simulink model "Channelizer"  (R2023a)
settings: Solver=VariableStepAuto  StartTime=0.0  StopTime=inf  RelTol=1e-3
InitFcn:
  | init;
values from neighbouring files (symbols this model uses):
  ch0_en = 0    [init.m]
  ch0_qam = 0    [init.m]
  ch0_swp = 0    [init.m]
  ch10_en = 0    [init.m]
  ch10_qam = 0    [init.m]
  ch10_swp = 0    [init.m]
  ch11_en = 0    [init.m]
  ch11_qam = 0    [init.m]
  ch11_swp = 0    [init.m]
  ch12_en = 0    [init.m]
  ch12_qam = 0    [init.m]
  ch12_swp = 0    [init.m]
  ch13_en = 0    [init.m]
  ch13_qam = 0    [init.m]
  ch13_swp = 0    [init.m]
  ch14_en = 0    [init.m]
  ch14_qam = 0    [init.m]
  ch14_swp = 0    [init.m]
  ch15_en = 0    [init.m]
  ch15_qam = 0    [init.m]
  ch15_swp = 0    [init.m]
  ch1_en = 1    [init.m]
  ch1_qam = 0    [init.m]
  ch1_swp = 0    [init.m]
  ch2_en = 1    [init.m]
  ch2_qam = 0    [init.m]
  ch2_swp = 0    [init.m]
  ch3_en = 0    [init.m]
  ch3_qam = 0    [init.m]
  ch3_swp = 0    [init.m]
  ch4_en = 0    [init.m]
  ch4_qam = 0    [init.m]
  ch4_swp = 0    [init.m]
  ch5_en = 1    [init.m]
  ch5_qam = 1    [init.m]
  ch5_swp = 0    [init.m]
  ch6_en = 1    [init.m]
  ch6_qam = 1    [init.m]
  ch6_swp = 0    [init.m]
  ch7_en = 0    [init.m]
  ch7_qam = 0    [init.m]
  ch7_swp = 0    [init.m]
  ch8_en = 0    [init.m]
  ch8_qam = 0    [init.m]
  ch8_swp = 0    [init.m]
  ch9_en = 0    [init.m]
  ch9_qam = 0    [init.m]
  ch9_swp = 0    [init.m]
  ch_filt_coef = 28 * ch_filt_coef / sum(ch_filt_coef(:))    [init.m]
  N = 512    [init.m]
  spec1_ch = 1    [init.m]
  spec2_ch = 2    [init.m]
  spec3_ch = 5    [init.m]
  spec4_ch = 6    [init.m]
  swp_rate0 = 0    [init.m]
  swp_rate1 = 0    [init.m]
  swp_rate10 = 0    [init.m]
  swp_rate11 = 0    [init.m]
  swp_rate12 = 0    [init.m]
  swp_rate13 = 0    [init.m]
  swp_rate14 = 0    [init.m]
  swp_rate15 = 0    [init.m]
  swp_rate2 = 0    [init.m]
  swp_rate3 = 0    [init.m]
  swp_rate4 = 0    [init.m]
  swp_rate5 = 0    [init.m]
  swp_rate6 = 0    [init.m]
  swp_rate7 = 0    [init.m]
  swp_rate8 = 0    [init.m]
  swp_rate9 = 0    [init.m]
  Ts = 16*(7/4)/8.75e9    (= 3.2e-09)    [init.m]
undefined symbols (not defined in the file or in its folder): S, vsva2197, xcvc1902
libraries: aieBasic x56, aieUtilities x47, dspswit3 x16, dspsigops x16, hlsBasic x3, dspindex x1, vmcUtilities x1, commchan3 x1
(part 4 of 4)

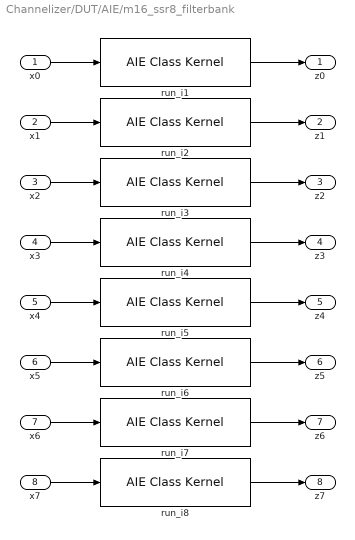
== system Channelizer/DUT/AIE/m16_ssr8_filterbank ==
  x0 : Inport
  x1 : Inport  Port=2
  x2 : Inport  Port=3
  x3 : Inport  Port=4
  x4 : Inport  Port=5
  x5 : Inport  Port=6
  x6 : Inport  Port=7
  x7 : Inport  Port=8
  run_i1 : aieBasic/AIE Class Kernel  KernelAllAttrs=|  PortNames={'sig_i'; 'sig_o'}  PortSerializedTypes={'{Q2{P{Tinput_stream{1{t{Scint16}}}}}}'; '{Q2{P{Toutput_stream{1{t{Scint16}}}}}}'}  PortWindowSizes={0.000000000000000000e+00; 0.000000000000000000e+00}  PortWindowMargins={0.000000000000000000e+00; 0.000000000000000000e+00}  PortSynchronicities={'auto', 'auto'}  PortSignalSizes={0.000000000000000000e+00; 2.048000000000000000e+03}  ClassTemplateSpecKind=implicit  ClassTemplateParamNames={'pattern'; 'NSAMP'}  ClassTemplateParamKinds={'nontype'; 'nontype'}  ClassTemplateParamTypes={'unsigned int'; 'unsigned int'}  ClassTemplateParamValues={'0', '2048'}  ClassCtorParamNames={'taps0_i'; 'taps1_i'}  ClassCtorParamSerializedTypes={'{R{C{Bi16}64}}'; '{R{C{Bi16}64}}'}  ClassCtorParamValues={'[0;2;-4;6;-13;54;-178;1985;-20;88;-287;1822;-22;100;-326;1570;2042;6;-4;2;259;-80;23;-8;569;-166;49;-9;911;-248;74;-14;-19;93;-307;1256;-14;74;-248;911;-9;49;-166;569;-8;23;-80;259;1256;-307;93;-19;1570;-326;100;-22;1822;-287;88;-20;1985;-178;54;-13]', '[6;12;-40;124;-6;28;-95;2027;-17;74;-241;1916;-22;97;-314;1706;2027;-95;28;-6;124;-40;12;6;408;-123;36;-8;737;-209;62;-12;-21;99;-322;1419;-17;85;-281;1085;-12;62;-209;737;-8;36;-123;408;1085;-281;85;-17;1419;-322;99;-21;1706;-314;97;-22;1916;-241;74;-17]'}  ClassIndex=1  ClassCtorIndex=1  ClassTabVisible=on  ClassTemplateParamsVisible=on  ClassCtorDeclVisible=on  ClassCtorParamsVisible=on  FunctionTabVisible=on  FunctionDecl=|  PortAttrs={ 'input', 'sig_i', 'input_stream_cint16 * restrict', '', '', '', ''; 'output', 'sig_o', 'output_stream_cint16 * restrict', '', '', '', '4*N' }  PortAttrsEnables={'off', 'off', 'off', 'off', 'off', 'off', 'off';'off', 'off', 'off', 'off', 'off', 'off', 'on'}  SampleTime=-1  ClassDeclTypeOptions=C[1 1]@t74@template < unsigned int pattern, unsigned int NSAMP > class polyphase_fir;  ClassDecl=template < unsigned int pattern, unsigned int NSAMP > class polyphase_fir;  ClassTemplateParams={ 'pattern', 'unsigned int', '0'; 'NSAMP', 'unsigned int', '4*N' }  ClassTemplateParamsEnables={'off', 'off', 'on';'off', 'off', 'on'}  ClassCtorDeclTypeOptions=C[1 1]@t69@polyphase_fir(int16 ( & taps0_i ) [ 64 ], int16 ( & taps1_i ) [ 64 ])  ClassCtorDecl=polyphase_fir(int16 ( & taps0_i ) [ 64 ], int16 ( & taps1_i ) [ 64 ])  ClassCtorParams={ 'taps0_i', 'int16 ( &) [ 64 ]', 'tile0_tapsA'; 'taps1_i', 'int16 ( &) [ 64 ]', 'tile0_tapsB' }  KernelHeaderFile=aie/polyphase_fir.h  KernelClassName=polyphase_fir  KernelFunction=run_i  KernelSourceFile=aie/polyphase_fir.cpp  KernelSearchPaths={}  PreProcOptions={}  blockJsonConstraints=[]
      KernelAllAttrs=|
      | s[12;12;9;9;19;14;21;23;21;23;24;21;15;17;12;24;26;26;26;27;28;9;21;23;23;23;24;25;14;19;19;29]@FunctionNameDeclFileNamePortNamesPortTypesPortSerializedTypesPortDirectionsPortWindowSizeEnablesPortWindowMarginEnablesPortBufferSizeEnablesPortBufferMarginEnablesPortSynchronicityEnablesPortSignalSizeEnablesPortBufferSizesPortBufferMarginsFunctionDeclFunctionTemplateSpecKindFunctionTemplateParamNamesFunctionTemplateParamKindsFunctionTemplateParamTypesFunctionTemplateParamValuesFunctionTemplateParamEnablesClassDeclClassTemplateSpecKindClassTemplateParamNamesClassTemplateParamKindsClassTemplateParamTypesClassTemplateParamValuesClassTemplateParamEnablesClassCtorDeclsClassCtorParamNamesClassCtorParamTypesClassCtorParamSerializedTypes[1 1]@C[32 1]@t5@run_it25@../../aie/polyphase_fir.hC[2 1]@t5@sig_it5@sig_oC[2 1]@t30@input_stream_cint16 * restrictt31@output_stream_cint16 * restrictC[2 1]@t37@{Q2{P{Tinput_stream{1{t{Scint16}}}}}}t38@{Q2{P{Toutput_stream{1{t{Scint16}}}}}}C[2 1]@t5@inputt6@outputC[2 1]@l0@l0@C[2 1]@l0@l0@C[2 1]@l0@l0@C[2 1]@l0@l0@C[2 1]@l0@l0@C[2 1]@l0@l1@C[2 1]@nnC[2 1]@nnt158@template < unsigned int pattern, unsigned int NSAMP > 
      | void polyphase_fir::
      | run_i(input_stream_cint16 * restrict sig_i, output_stream_cint16 * restrict sig_o)t4@nonee[0 1]@e[0 1]@e[0 1]@e[0 1]@e[0 1]@t74@template < unsigned int pattern, unsigned int NSAMP > class polyphase_fir;t8@implicitC[2 1]@t7@patternt5@NSAMPC[2 1]@t7@nontypet7@nontypeC[2 1]@t12@unsigned intt12@unsigned intC[2 1]@nnC[2 1]@l1@l1@C[1 1]@t69@polyphase_fir(int16 ( & taps0_i ) [ 64 ], int16 ( & taps1_i ) [ 64 ])C[1 1]@C[2 1]@t7@taps0_it7@taps1_iC[1 1]@C[2 1]@t17@int16 ( &) [ 64 ]t17@int16 ( &) [ 64 ]C[1 1]@C[2 1]@t14@{R{C{Bi16}64}}t14@{R{C{Bi16}64}}
      FunctionDecl=|
      | template < unsigned int pattern, unsigned int NSAMP > 
      | void polyphase_fir::
      | run_i(input_stream_cint16 * restrict sig_i, output_stream_cint16 * restrict sig_o)
  run_i2 : aieBasic/AIE Class Kernel  KernelAllAttrs=|  PortNames={'sig_i'; 'sig_o'}  PortSerializedTypes={'{Q2{P{Tinput_stream{1{t{Scint16}}}}}}'; '{Q2{P{Toutput_stream{1{t{Scint16}}}}}}'}  PortWindowSizes={0.000000000000000000e+00; 0.000000000000000000e+00}  PortWindowMargins={0.000000000000000000e+00; 0.000000000000000000e+00}  PortSynchronicities={'auto', 'auto'}  PortSignalSizes={0.000000000000000000e+00; 2.048000000000000000e+03}  ClassTemplateSpecKind=implicit  ClassTemplateParamNames={'pattern'; 'NSAMP'}  ClassTemplateParamKinds={'nontype'; 'nontype'}  ClassTemplateParamTypes={'unsigned int'; 'unsigned int'}  ClassTemplateParamValues={'1', '2048'}  ClassCtorParamNames={'taps0_i'; 'taps1_i'}  ClassCtorParamSerializedTypes={'{R{C{Bi16}64}}'; '{R{C{Bi16}64}}'}  ClassCtorParamValues={'[-8;23;-80;259;0;2;-4;6;-13;54;-178;1985;-20;88;-287;1822;1985;-178;54;-13;2042;6;-4;2;259;-80;23;-8;569;-166;49;-9;-22;100;-326;1570;-19;93;-307;1256;-14;74;-248;911;-9;49;-166;569;911;-248;74;-14;1256;-307;93;-19;1570;-326;100;-22;1822;-287;88;-20]', '[-8;36;-123;408;6;12;-40;124;-6;28;-95;2027;-17;74;-241;1916;1916;-241;74;-17;2027;-95;28;-6;124;-40;12;6;408;-123;36;-8;-22;97;-314;1706;-21;99;-322;1419;-17;85;-281;1085;-12;62;-209;737;737;-209;62;-12;1085;-281;85;-17;1419;-322;99;-21;1706;-314;97;-22]'}  ClassIndex=1  ClassCtorIndex=1  ClassTabVisible=on  ClassTemplateParamsVisible=on  ClassCtorDeclVisible=on  ClassCtorParamsVisible=on  FunctionTabVisible=on  FunctionDecl=|  PortAttrs={ 'input', 'sig_i', 'input_stream_cint16 * restrict', '', '', '', ''; 'output', 'sig_o', 'output_stream_cint16 * restrict', '', '', '', '4*N' }  PortAttrsEnables={'off', 'off', 'off', 'off', 'off', 'off', 'off';'off', 'off', 'off', 'off', 'off', 'off', 'on'}  SampleTime=-1  ClassDeclTypeOptions=C[1 1]@t74@template < unsigned int pattern, unsigned int NSAMP > class polyphase_fir;  ClassDecl=template < unsigned int pattern, unsigned int NSAMP > class polyphase_fir;  ClassTemplateParams={ 'pattern', 'unsigned int', '1'; 'NSAMP', 'unsigned int', '4*N' }  ClassTemplateParamsEnables={'off', 'off', 'on';'off', 'off', 'on'}  ClassCtorDeclTypeOptions=C[1 1]@t69@polyphase_fir(int16 ( & taps0_i ) [ 64 ], int16 ( & taps1_i ) [ 64 ])  ClassCtorDecl=polyphase_fir(int16 ( & taps0_i ) [ 64 ], int16 ( & taps1_i ) [ 64 ])  ClassCtorParams={ 'taps0_i', 'int16 ( &) [ 64 ]', 'tile1_tapsA'; 'taps1_i', 'int16 ( &) [ 64 ]', 'tile1_tapsB' }  KernelHeaderFile=aie/polyphase_fir.h  KernelClassName=polyphase_fir  KernelFunction=run_i  KernelSourceFile=aie/polyphase_fir.cpp  KernelSearchPaths={}  PreProcOptions={}  blockJsonConstraints=[]
      KernelAllAttrs=|
      | s[12;12;9;9;19;14;21;23;21;23;24;21;15;17;12;24;26;26;26;27;28;9;21;23;23;23;24;25;14;19;19;29]@FunctionNameDeclFileNamePortNamesPortTypesPortSerializedTypesPortDirectionsPortWindowSizeEnablesPortWindowMarginEnablesPortBufferSizeEnablesPortBufferMarginEnablesPortSynchronicityEnablesPortSignalSizeEnablesPortBufferSizesPortBufferMarginsFunctionDeclFunctionTemplateSpecKindFunctionTemplateParamNamesFunctionTemplateParamKindsFunctionTemplateParamTypesFunctionTemplateParamValuesFunctionTemplateParamEnablesClassDeclClassTemplateSpecKindClassTemplateParamNamesClassTemplateParamKindsClassTemplateParamTypesClassTemplateParamValuesClassTemplateParamEnablesClassCtorDeclsClassCtorParamNamesClassCtorParamTypesClassCtorParamSerializedTypes[1 1]@C[32 1]@t5@run_it25@../../aie/polyphase_fir.hC[2 1]@t5@sig_it5@sig_oC[2 1]@t30@input_stream_cint16 * restrictt31@output_stream_cint16 * restrictC[2 1]@t37@{Q2{P{Tinput_stream{1{t{Scint16}}}}}}t38@{Q2{P{Toutput_stream{1{t{Scint16}}}}}}C[2 1]@t5@inputt6@outputC[2 1]@l0@l0@C[2 1]@l0@l0@C[2 1]@l0@l0@C[2 1]@l0@l0@C[2 1]@l0@l0@C[2 1]@l0@l1@C[2 1]@nnC[2 1]@nnt158@template < unsigned int pattern, unsigned int NSAMP > 
      | void polyphase_fir::
      | run_i(input_stream_cint16 * restrict sig_i, output_stream_cint16 * restrict sig_o)t4@nonee[0 1]@e[0 1]@e[0 1]@e[0 1]@e[0 1]@t74@template < unsigned int pattern, unsigned int NSAMP > class polyphase_fir;t8@implicitC[2 1]@t7@patternt5@NSAMPC[2 1]@t7@nontypet7@nontypeC[2 1]@t12@unsigned intt12@unsigned intC[2 1]@nnC[2 1]@l1@l1@C[1 1]@t69@polyphase_fir(int16 ( & taps0_i ) [ 64 ], int16 ( & taps1_i ) [ 64 ])C[1 1]@C[2 1]@t7@taps0_it7@taps1_iC[1 1]@C[2 1]@t17@int16 ( &) [ 64 ]t17@int16 ( &) [ 64 ]C[1 1]@C[2 1]@t14@{R{C{Bi16}64}}t14@{R{C{Bi16}64}}
      FunctionDecl=|
      | template < unsigned int pattern, unsigned int NSAMP > 
      | void polyphase_fir::
      | run_i(input_stream_cint16 * restrict sig_i, output_stream_cint16 * restrict sig_o)
  run_i3 : aieBasic/AIE Class Kernel  KernelAllAttrs=|  PortNames={'sig_i'; 'sig_o'}  PortSerializedTypes={'{Q2{P{Tinput_stream{1{t{Scint16}}}}}}'; '{Q2{P{Toutput_stream{1{t{Scint16}}}}}}'}  PortWindowSizes={0.000000000000000000e+00; 0.000000000000000000e+00}  PortWindowMargins={0.000000000000000000e+00; 0.000000000000000000e+00}  PortSynchronicities={'auto', 'auto'}  PortSignalSizes={0.000000000000000000e+00; 2.048000000000000000e+03}  ClassTemplateSpecKind=implicit  ClassTemplateParamNames={'pattern'; 'NSAMP'}  ClassTemplateParamKinds={'nontype'; 'nontype'}  ClassTemplateParamTypes={'unsigned int'; 'unsigned int'}  ClassTemplateParamValues={'2', '2048'}  ClassCtorParamNames={'taps0_i'; 'taps1_i'}  ClassCtorParamSerializedTypes={'{R{C{Bi16}64}}'; '{R{C{Bi16}64}}'}  ClassCtorParamValues={'[-9;49;-166;569;-8;23;-80;259;0;2;-4;6;-13;54;-178;1985;1822;-287;88;-20;1985;-178;54;-13;2042;6;-4;2;259;-80;23;-8;-20;88;-287;1822;-22;100;-326;1570;-19;93;-307;1256;-14;74;-248;911;569;-166;49;-9;911;-248;74;-14;1256;-307;93;-19;1570;-326;100;-22]', '[-12;62;-209;737;-8;36;-123;408;6;12;-40;124;-6;28;-95;2027;1706;-314;97;-22;1916;-241;74;-17;2027;-95;28;-6;124;-40;12;6;-17;74;-241;1916;-22;97;-314;1706;-21;99;-322;1419;-17;85;-281;1085;408;-123;36;-8;737;-209;62;-12;1085;-281;85;-17;1419;-322;99;-21]'}  ClassIndex=1  ClassCtorIndex=1  ClassTabVisible=on  ClassTemplateParamsVisible=on  ClassCtorDeclVisible=on  ClassCtorParamsVisible=on  FunctionTabVisible=on  FunctionDecl=|  PortAttrs={ 'input', 'sig_i', 'input_stream_cint16 * restrict', '', '', '', ''; 'output', 'sig_o', 'output_stream_cint16 * restrict', '', '', '', '4*N' }  PortAttrsEnables={'off', 'off', 'off', 'off', 'off', 'off', 'off';'off', 'off', 'off', 'off', 'off', 'off', 'on'}  SampleTime=-1  ClassDeclTypeOptions=C[1 1]@t74@template < unsigned int pattern, unsigned int NSAMP > class polyphase_fir;  ClassDecl=template < unsigned int pattern, unsigned int NSAMP > class polyphase_fir;  ClassTemplateParams={ 'pattern', 'unsigned int', '2'; 'NSAMP', 'unsigned int', '4*N' }  ClassTemplateParamsEnables={'off', 'off', 'on';'off', 'off', 'on'}  ClassCtorDeclTypeOptions=C[1 1]@t69@polyphase_fir(int16 ( & taps0_i ) [ 64 ], int16 ( & taps1_i ) [ 64 ])  ClassCtorDecl=polyphase_fir(int16 ( & taps0_i ) [ 64 ], int16 ( & taps1_i ) [ 64 ])  ClassCtorParams={ 'taps0_i', 'int16 ( &) [ 64 ]', 'tile2_tapsA'; 'taps1_i', 'int16 ( &) [ 64 ]', 'tile2_tapsB' }  KernelHeaderFile=aie/polyphase_fir.h  KernelClassName=polyphase_fir  KernelFunction=run_i  KernelSourceFile=aie/polyphase_fir.cpp  KernelSearchPaths={}  PreProcOptions={}  blockJsonConstraints=[]
      KernelAllAttrs=|
      | s[12;12;9;9;19;14;21;23;21;23;24;21;15;17;12;24;26;26;26;27;28;9;21;23;23;23;24;25;14;19;19;29]@FunctionNameDeclFileNamePortNamesPortTypesPortSerializedTypesPortDirectionsPortWindowSizeEnablesPortWindowMarginEnablesPortBufferSizeEnablesPortBufferMarginEnablesPortSynchronicityEnablesPortSignalSizeEnablesPortBufferSizesPortBufferMarginsFunctionDeclFunctionTemplateSpecKindFunctionTemplateParamNamesFunctionTemplateParamKindsFunctionTemplateParamTypesFunctionTemplateParamValuesFunctionTemplateParamEnablesClassDeclClassTemplateSpecKindClassTemplateParamNamesClassTemplateParamKindsClassTemplateParamTypesClassTemplateParamValuesClassTemplateParamEnablesClassCtorDeclsClassCtorParamNamesClassCtorParamTypesClassCtorParamSerializedTypes[1 1]@C[32 1]@t5@run_it25@../../aie/polyphase_fir.hC[2 1]@t5@sig_it5@sig_oC[2 1]@t30@input_stream_cint16 * restrictt31@output_stream_cint16 * restrictC[2 1]@t37@{Q2{P{Tinput_stream{1{t{Scint16}}}}}}t38@{Q2{P{Toutput_stream{1{t{Scint16}}}}}}C[2 1]@t5@inputt6@outputC[2 1]@l0@l0@C[2 1]@l0@l0@C[2 1]@l0@l0@C[2 1]@l0@l0@C[2 1]@l0@l0@C[2 1]@l0@l1@C[2 1]@nnC[2 1]@nnt158@template < unsigned int pattern, unsigned int NSAMP > 
      | void polyphase_fir::
      | run_i(input_stream_cint16 * restrict sig_i, output_stream_cint16 * restrict sig_o)t4@nonee[0 1]@e[0 1]@e[0 1]@e[0 1]@e[0 1]@t74@template < unsigned int pattern, unsigned int NSAMP > class polyphase_fir;t8@implicitC[2 1]@t7@patternt5@NSAMPC[2 1]@t7@nontypet7@nontypeC[2 1]@t12@unsigned intt12@unsigned intC[2 1]@nnC[2 1]@l1@l1@C[1 1]@t69@polyphase_fir(int16 ( & taps0_i ) [ 64 ], int16 ( & taps1_i ) [ 64 ])C[1 1]@C[2 1]@t7@taps0_it7@taps1_iC[1 1]@C[2 1]@t17@int16 ( &) [ 64 ]t17@int16 ( &) [ 64 ]C[1 1]@C[2 1]@t14@{R{C{Bi16}64}}t14@{R{C{Bi16}64}}
      FunctionDecl=|
      | template < unsigned int pattern, unsigned int NSAMP > 
      | void polyphase_fir::
      | run_i(input_stream_cint16 * restrict sig_i, output_stream_cint16 * restrict sig_o)
  run_i4 : aieBasic/AIE Class Kernel  KernelAllAttrs=|  PortNames={'sig_i'; 'sig_o'}  PortSerializedTypes={'{Q2{P{Tinput_stream{1{t{Scint16}}}}}}'; '{Q2{P{Toutput_stream{1{t{Scint16}}}}}}'}  PortWindowSizes={0.000000000000000000e+00; 0.000000000000000000e+00}  PortWindowMargins={0.000000000000000000e+00; 0.000000000000000000e+00}  PortSynchronicities={'auto', 'auto'}  PortSignalSizes={0.000000000000000000e+00; 2.048000000000000000e+03}  ClassTemplateSpecKind=implicit  ClassTemplateParamNames={'pattern'; 'NSAMP'}  ClassTemplateParamKinds={'nontype'; 'nontype'}  ClassTemplateParamTypes={'unsigned int'; 'unsigned int'}  ClassTemplateParamValues={'3', '2048'}  ClassCtorParamNames={'taps0_i'; 'taps1_i'}  ClassCtorParamSerializedTypes={'{R{C{Bi16}64}}'; '{R{C{Bi16}64}}'}  ClassCtorParamValues={'[-14;74;-248;911;-9;49;-166;569;-8;23;-80;259;0;2;-4;6;1570;-326;100;-22;1822;-287;88;-20;1985;-178;54;-13;2042;6;-4;2;-13;54;-178;1985;-20;88;-287;1822;-22;100;-326;1570;-19;93;-307;1256;259;-80;23;-8;569;-166;49;-9;911;-248;74;-14;1256;-307;93;-19]', '[-17;85;-281;1085;-12;62;-209;737;-8;36;-123;408;6;12;-40;124;1419;-322;99;-21;1706;-314;97;-22;1916;-241;74;-17;2027;-95;28;-6;-6;28;-95;2027;-17;74;-241;1916;-22;97;-314;1706;-21;99;-322;1419;124;-40;12;6;408;-123;36;-8;737;-209;62;-12;1085;-281;85;-17]'}  ClassIndex=1  ClassCtorIndex=1  ClassTabVisible=on  ClassTemplateParamsVisible=on  ClassCtorDeclVisible=on  ClassCtorParamsVisible=on  FunctionTabVisible=on  FunctionDecl=|  PortAttrs={ 'input', 'sig_i', 'input_stream_cint16 * restrict', '', '', '', ''; 'output', 'sig_o', 'output_stream_cint16 * restrict', '', '', '', '4*N' }  PortAttrsEnables={'off', 'off', 'off', 'off', 'off', 'off', 'off';'off', 'off', 'off', 'off', 'off', 'off', 'on'}  SampleTime=-1  ClassDeclTypeOptions=C[1 1]@t74@template < unsigned int pattern, unsigned int NSAMP > class polyphase_fir;  ClassDecl=template < unsigned int pattern, unsigned int NSAMP > class polyphase_fir;  ClassTemplateParams={ 'pattern', 'unsigned int', '3'; 'NSAMP', 'unsigned int', '4*N' }  ClassTemplateParamsEnables={'off', 'off', 'on';'off', 'off', 'on'}  ClassCtorDeclTypeOptions=C[1 1]@t69@polyphase_fir(int16 ( & taps0_i ) [ 64 ], int16 ( & taps1_i ) [ 64 ])  ClassCtorDecl=polyphase_fir(int16 ( & taps0_i ) [ 64 ], int16 ( & taps1_i ) [ 64 ])  ClassCtorParams={ 'taps0_i', 'int16 ( &) [ 64 ]', 'tile3_tapsA'; 'taps1_i', 'int16 ( &) [ 64 ]', 'tile3_tapsB' }  KernelHeaderFile=aie/polyphase_fir.h  KernelClassName=polyphase_fir  KernelFunction=run_i  KernelSourceFile=aie/polyphase_fir.cpp  KernelSearchPaths={}  PreProcOptions={}  blockJsonConstraints=[]
      KernelAllAttrs=|
      | s[12;12;9;9;19;14;21;23;21;23;24;21;15;17;12;24;26;26;26;27;28;9;21;23;23;23;24;25;14;19;19;29]@FunctionNameDeclFileNamePortNamesPortTypesPortSerializedTypesPortDirectionsPortWindowSizeEnablesPortWindowMarginEnablesPortBufferSizeEnablesPortBufferMarginEnablesPortSynchronicityEnablesPortSignalSizeEnablesPortBufferSizesPortBufferMarginsFunctionDeclFunctionTemplateSpecKindFunctionTemplateParamNamesFunctionTemplateParamKindsFunctionTemplateParamTypesFunctionTemplateParamValuesFunctionTemplateParamEnablesClassDeclClassTemplateSpecKindClassTemplateParamNamesClassTemplateParamKindsClassTemplateParamTypesClassTemplateParamValuesClassTemplateParamEnablesClassCtorDeclsClassCtorParamNamesClassCtorParamTypesClassCtorParamSerializedTypes[1 1]@C[32 1]@t5@run_it25@../../aie/polyphase_fir.hC[2 1]@t5@sig_it5@sig_oC[2 1]@t30@input_stream_cint16 * restrictt31@output_stream_cint16 * restrictC[2 1]@t37@{Q2{P{Tinput_stream{1{t{Scint16}}}}}}t38@{Q2{P{Toutput_stream{1{t{Scint16}}}}}}C[2 1]@t5@inputt6@outputC[2 1]@l0@l0@C[2 1]@l0@l0@C[2 1]@l0@l0@C[2 1]@l0@l0@C[2 1]@l0@l0@C[2 1]@l0@l1@C[2 1]@nnC[2 1]@nnt158@template < unsigned int pattern, unsigned int NSAMP > 
      | void polyphase_fir::
      | run_i(input_stream_cint16 * restrict sig_i, output_stream_cint16 * restrict sig_o)t4@nonee[0 1]@e[0 1]@e[0 1]@e[0 1]@e[0 1]@t74@template < unsigned int pattern, unsigned int NSAMP > class polyphase_fir;t8@implicitC[2 1]@t7@patternt5@NSAMPC[2 1]@t7@nontypet7@nontypeC[2 1]@t12@unsigned intt12@unsigned intC[2 1]@nnC[2 1]@l1@l1@C[1 1]@t69@polyphase_fir(int16 ( & taps0_i ) [ 64 ], int16 ( & taps1_i ) [ 64 ])C[1 1]@C[2 1]@t7@taps0_it7@taps1_iC[1 1]@C[2 1]@t17@int16 ( &) [ 64 ]t17@int16 ( &) [ 64 ]C[1 1]@C[2 1]@t14@{R{C{Bi16}64}}t14@{R{C{Bi16}64}}
      FunctionDecl=|
      | template < unsigned int pattern, unsigned int NSAMP > 
      | void polyphase_fir::
      | run_i(input_stream_cint16 * restrict sig_i, output_stream_cint16 * restrict sig_o)
  run_i5 : aieBasic/AIE Class Kernel  KernelAllAttrs=|  PortNames={'sig_i'; 'sig_o'}  PortSerializedTypes={'{Q2{P{Tinput_stream{1{t{Scint16}}}}}}'; '{Q2{P{Toutput_stream{1{t{Scint16}}}}}}'}  PortWindowSizes={0.000000000000000000e+00; 0.000000000000000000e+00}  PortWindowMargins={0.000000000000000000e+00; 0.000000000000000000e+00}  PortSynchronicities={'auto', 'auto'}  PortSignalSizes={0.000000000000000000e+00; 2.048000000000000000e+03}  ClassTemplateSpecKind=implicit  ClassTemplateParamNames={'pattern'; 'NSAMP'}  ClassTemplateParamKinds={'nontype'; 'nontype'}  ClassTemplateParamTypes={'unsigned int'; 'unsigned int'}  ClassTemplateParamValues={'4', '2048'}  ClassCtorParamNames={'taps0_i'; 'taps1_i'}  ClassCtorParamSerializedTypes={'{R{C{Bi16}64}}'; '{R{C{Bi16}64}}'}  ClassCtorParamValues={'[-19;93;-307;1256;-14;74;-248;911;-9;49;-166;569;-8;23;-80;259;1256;-307;93;-19;1570;-326;100;-22;1822;-287;88;-20;1985;-178;54;-13;0;2;-4;6;-13;54;-178;1985;-20;88;-287;1822;-22;100;-326;1570;2042;6;-4;2;259;-80;23;-8;569;-166;49;-9;911;-248;74;-14]', '[-21;99;-322;1419;-17;85;-281;1085;-12;62;-209;737;-8;36;-123;408;1085;-281;85;-17;1419;-322;99;-21;1706;-314;97;-22;1916;-241;74;-17;6;12;-40;124;-6;28;-95;2027;-17;74;-241;1916;-22;97;-314;1706;2027;-95;28;-6;124;-40;12;6;408;-123;36;-8;737;-209;62;-12]'}  ClassIndex=1  ClassCtorIndex=1  ClassTabVisible=on  ClassTemplateParamsVisible=on  ClassCtorDeclVisible=on  ClassCtorParamsVisible=on  FunctionTabVisible=on  FunctionDecl=|  PortAttrs={ 'input', 'sig_i', 'input_stream_cint16 * restrict', '', '', '', ''; 'output', 'sig_o', 'output_stream_cint16 * restrict', '', '', '', '4*N' }  PortAttrsEnables={'off', 'off', 'off', 'off', 'off', 'off', 'off';'off', 'off', 'off', 'off', 'off', 'off', 'on'}  SampleTime=-1  ClassDeclTypeOptions=C[1 1]@t74@template < unsigned int pattern, unsigned int NSAMP > class polyphase_fir;  ClassDecl=template < unsigned int pattern, unsigned int NSAMP > class polyphase_fir;  ClassTemplateParams={ 'pattern', 'unsigned int', '4'; 'NSAMP', 'unsigned int', '4*N' }  ClassTemplateParamsEnables={'off', 'off', 'on';'off', 'off', 'on'}  ClassCtorDeclTypeOptions=C[1 1]@t69@polyphase_fir(int16 ( & taps0_i ) [ 64 ], int16 ( & taps1_i ) [ 64 ])  ClassCtorDecl=polyphase_fir(int16 ( & taps0_i ) [ 64 ], int16 ( & taps1_i ) [ 64 ])  ClassCtorParams={ 'taps0_i', 'int16 ( &) [ 64 ]', 'tile4_tapsA'; 'taps1_i', 'int16 ( &) [ 64 ]', 'tile4_tapsB' }  KernelHeaderFile=aie/polyphase_fir.h  KernelClassName=polyphase_fir  KernelFunction=run_i  KernelSourceFile=aie/polyphase_fir.cpp  KernelSearchPaths={}  PreProcOptions={}  blockJsonConstraints=[]
      KernelAllAttrs=|
      | s[12;12;9;9;19;14;21;23;21;23;24;21;15;17;12;24;26;26;26;27;28;9;21;23;23;23;24;25;14;19;19;29]@FunctionNameDeclFileNamePortNamesPortTypesPortSerializedTypesPortDirectionsPortWindowSizeEnablesPortWindowMarginEnablesPortBufferSizeEnablesPortBufferMarginEnablesPortSynchronicityEnablesPortSignalSizeEnablesPortBufferSizesPortBufferMarginsFunctionDeclFunctionTemplateSpecKindFunctionTemplateParamNamesFunctionTemplateParamKindsFunctionTemplateParamTypesFunctionTemplateParamValuesFunctionTemplateParamEnablesClassDeclClassTemplateSpecKindClassTemplateParamNamesClassTemplateParamKindsClassTemplateParamTypesClassTemplateParamValuesClassTemplateParamEnablesClassCtorDeclsClassCtorParamNamesClassCtorParamTypesClassCtorParamSerializedTypes[1 1]@C[32 1]@t5@run_it25@../../aie/polyphase_fir.hC[2 1]@t5@sig_it5@sig_oC[2 1]@t30@input_stream_cint16 * restrictt31@output_stream_cint16 * restrictC[2 1]@t37@{Q2{P{Tinput_stream{1{t{Scint16}}}}}}t38@{Q2{P{Toutput_stream{1{t{Scint16}}}}}}C[2 1]@t5@inputt6@outputC[2 1]@l0@l0@C[2 1]@l0@l0@C[2 1]@l0@l0@C[2 1]@l0@l0@C[2 1]@l0@l0@C[2 1]@l0@l1@C[2 1]@nnC[2 1]@nnt158@template < unsigned int pattern, unsigned int NSAMP > 
      | void polyphase_fir::
      | run_i(input_stream_cint16 * restrict sig_i, output_stream_cint16 * restrict sig_o)t4@nonee[0 1]@e[0 1]@e[0 1]@e[0 1]@e[0 1]@t74@template < unsigned int pattern, unsigned int NSAMP > class polyphase_fir;t8@implicitC[2 1]@t7@patternt5@NSAMPC[2 1]@t7@nontypet7@nontypeC[2 1]@t12@unsigned intt12@unsigned intC[2 1]@nnC[2 1]@l1@l1@C[1 1]@t69@polyphase_fir(int16 ( & taps0_i ) [ 64 ], int16 ( & taps1_i ) [ 64 ])C[1 1]@C[2 1]@t7@taps0_it7@taps1_iC[1 1]@C[2 1]@t17@int16 ( &) [ 64 ]t17@int16 ( &) [ 64 ]C[1 1]@C[2 1]@t14@{R{C{Bi16}64}}t14@{R{C{Bi16}64}}
      FunctionDecl=|
      | template < unsigned int pattern, unsigned int NSAMP > 
      | void polyphase_fir::
      | run_i(input_stream_cint16 * restrict sig_i, output_stream_cint16 * restrict sig_o)
  run_i6 : aieBasic/AIE Class Kernel  KernelAllAttrs=|  PortNames={'sig_i'; 'sig_o'}  PortSerializedTypes={'{Q2{P{Tinput_stream{1{t{Scint16}}}}}}'; '{Q2{P{Toutput_stream{1{t{Scint16}}}}}}'}  PortWindowSizes={0.000000000000000000e+00; 0.000000000000000000e+00}  PortWindowMargins={0.000000000000000000e+00; 0.000000000000000000e+00}  PortSynchronicities={'auto', 'auto'}  PortSignalSizes={0.000000000000000000e+00; 2.048000000000000000e+03}  ClassTemplateSpecKind=implicit  ClassTemplateParamNames={'pattern'; 'NSAMP'}  ClassTemplateParamKinds={'nontype'; 'nontype'}  ClassTemplateParamTypes={'unsigned int'; 'unsigned int'}  ClassTemplateParamValues={'5', '2048'}  ClassCtorParamNames={'taps0_i'; 'taps1_i'}  ClassCtorParamSerializedTypes={'{R{C{Bi16}64}}'; '{R{C{Bi16}64}}'}  ClassCtorParamValues={'[-22;100;-326;1570;-19;93;-307;1256;-14;74;-248;911;-9;49;-166;569;911;-248;74;-14;1256;-307;93;-19;1570;-326;100;-22;1822;-287;88;-20;-8;23;-80;259;0;2;-4;6;-13;54;-178;1985;-20;88;-287;1822;1985;-178;54;-13;2042;6;-4;2;259;-80;23;-8;569;-166;49;-9]', '[-22;97;-314;1706;-21;99;-322;1419;-17;85;-281;1085;-12;62;-209;737;737;-209;62;-12;1085;-281;85;-17;1419;-322;99;-21;1706;-314;97;-22;-8;36;-123;408;6;12;-40;124;-6;28;-95;2027;-17;74;-241;1916;1916;-241;74;-17;2027;-95;28;-6;124;-40;12;6;408;-123;36;-8]'}  ClassIndex=1  ClassCtorIndex=1  ClassTabVisible=on  ClassTemplateParamsVisible=on  ClassCtorDeclVisible=on  ClassCtorParamsVisible=on  FunctionTabVisible=on  FunctionDecl=|  PortAttrs={ 'input', 'sig_i', 'input_stream_cint16 * restrict', '', '', '', ''; 'output', 'sig_o', 'output_stream_cint16 * restrict', '', '', '', '4*N' }  PortAttrsEnables={'off', 'off', 'off', 'off', 'off', 'off', 'off';'off', 'off', 'off', 'off', 'off', 'off', 'on'}  SampleTime=-1  ClassDeclTypeOptions=C[1 1]@t74@template < unsigned int pattern, unsigned int NSAMP > class polyphase_fir;  ClassDecl=template < unsigned int pattern, unsigned int NSAMP > class polyphase_fir;  ClassTemplateParams={ 'pattern', 'unsigned int', '5'; 'NSAMP', 'unsigned int', '4*N' }  ClassTemplateParamsEnables={'off', 'off', 'on';'off', 'off', 'on'}  ClassCtorDeclTypeOptions=C[1 1]@t69@polyphase_fir(int16 ( & taps0_i ) [ 64 ], int16 ( & taps1_i ) [ 64 ])  ClassCtorDecl=polyphase_fir(int16 ( & taps0_i ) [ 64 ], int16 ( & taps1_i ) [ 64 ])  ClassCtorParams={ 'taps0_i', 'int16 ( &) [ 64 ]', 'tile5_tapsA'; 'taps1_i', 'int16 ( &) [ 64 ]', 'tile5_tapsB' }  KernelHeaderFile=aie/polyphase_fir.h  KernelClassName=polyphase_fir  KernelFunction=run_i  KernelSourceFile=aie/polyphase_fir.cpp  KernelSearchPaths={}  PreProcOptions={}  blockJsonConstraints=[]
      KernelAllAttrs=|
      | s[12;12;9;9;19;14;21;23;21;23;24;21;15;17;12;24;26;26;26;27;28;9;21;23;23;23;24;25;14;19;19;29]@FunctionNameDeclFileNamePortNamesPortTypesPortSerializedTypesPortDirectionsPortWindowSizeEnablesPortWindowMarginEnablesPortBufferSizeEnablesPortBufferMarginEnablesPortSynchronicityEnablesPortSignalSizeEnablesPortBufferSizesPortBufferMarginsFunctionDeclFunctionTemplateSpecKindFunctionTemplateParamNamesFunctionTemplateParamKindsFunctionTemplateParamTypesFunctionTemplateParamValuesFunctionTemplateParamEnablesClassDeclClassTemplateSpecKindClassTemplateParamNamesClassTemplateParamKindsClassTemplateParamTypesClassTemplateParamValuesClassTemplateParamEnablesClassCtorDeclsClassCtorParamNamesClassCtorParamTypesClassCtorParamSerializedTypes[1 1]@C[32 1]@t5@run_it25@../../aie/polyphase_fir.hC[2 1]@t5@sig_it5@sig_oC[2 1]@t30@input_stream_cint16 * restrictt31@output_stream_cint16 * restrictC[2 1]@t37@{Q2{P{Tinput_stream{1{t{Scint16}}}}}}t38@{Q2{P{Toutput_stream{1{t{Scint16}}}}}}C[2 1]@t5@inputt6@outputC[2 1]@l0@l0@C[2 1]@l0@l0@C[2 1]@l0@l0@C[2 1]@l0@l0@C[2 1]@l0@l0@C[2 1]@l0@l1@C[2 1]@nnC[2 1]@nnt158@template < unsigned int pattern, unsigned int NSAMP > 
      | void polyphase_fir::
      | run_i(input_stream_cint16 * restrict sig_i, output_stream_cint16 * restrict sig_o)t4@nonee[0 1]@e[0 1]@e[0 1]@e[0 1]@e[0 1]@t74@template < unsigned int pattern, unsigned int NSAMP > class polyphase_fir;t8@implicitC[2 1]@t7@patternt5@NSAMPC[2 1]@t7@nontypet7@nontypeC[2 1]@t12@unsigned intt12@unsigned intC[2 1]@nnC[2 1]@l1@l1@C[1 1]@t69@polyphase_fir(int16 ( & taps0_i ) [ 64 ], int16 ( & taps1_i ) [ 64 ])C[1 1]@C[2 1]@t7@taps0_it7@taps1_iC[1 1]@C[2 1]@t17@int16 ( &) [ 64 ]t17@int16 ( &) [ 64 ]C[1 1]@C[2 1]@t14@{R{C{Bi16}64}}t14@{R{C{Bi16}64}}
      FunctionDecl=|
      | template < unsigned int pattern, unsigned int NSAMP > 
      | void polyphase_fir::
      | run_i(input_stream_cint16 * restrict sig_i, output_stream_cint16 * restrict sig_o)
  run_i7 : aieBasic/AIE Class Kernel  KernelAllAttrs=|  PortNames={'sig_i'; 'sig_o'}  PortSerializedTypes={'{Q2{P{Tinput_stream{1{t{Scint16}}}}}}'; '{Q2{P{Toutput_stream{1{t{Scint16}}}}}}'}  PortWindowSizes={0.000000000000000000e+00; 0.000000000000000000e+00}  PortWindowMargins={0.000000000000000000e+00; 0.000000000000000000e+00}  PortSynchronicities={'auto', 'auto'}  PortSignalSizes={0.000000000000000000e+00; 2.048000000000000000e+03}  ClassTemplateSpecKind=implicit  ClassTemplateParamNames={'pattern'; 'NSAMP'}  ClassTemplateParamKinds={'nontype'; 'nontype'}  ClassTemplateParamTypes={'unsigned int'; 'unsigned int'}  ClassTemplateParamValues={'6', '2048'}  ClassCtorParamNames={'taps0_i'; 'taps1_i'}  ClassCtorParamSerializedTypes={'{R{C{Bi16}64}}'; '{R{C{Bi16}64}}'}  ClassCtorParamValues={'[-20;88;-287;1822;-22;100;-326;1570;-19;93;-307;1256;-14;74;-248;911;569;-166;49;-9;911;-248;74;-14;1256;-307;93;-19;1570;-326;100;-22;-9;49;-166;569;-8;23;-80;259;0;2;-4;6;-13;54;-178;1985;1822;-287;88;-20;1985;-178;54;-13;2042;6;-4;2;259;-80;23;-8]', '[-17;74;-241;1916;-22;97;-314;1706;-21;99;-322;1419;-17;85;-281;1085;408;-123;36;-8;737;-209;62;-12;1085;-281;85;-17;1419;-322;99;-21;-12;62;-209;737;-8;36;-123;408;6;12;-40;124;-6;28;-95;2027;1706;-314;97;-22;1916;-241;74;-17;2027;-95;28;-6;124;-40;12;6]'}  ClassIndex=1  ClassCtorIndex=1  ClassTabVisible=on  ClassTemplateParamsVisible=on  ClassCtorDeclVisible=on  ClassCtorParamsVisible=on  FunctionTabVisible=on  FunctionDecl=|  PortAttrs={ 'input', 'sig_i', 'input_stream_cint16 * restrict', '', '', '', ''; 'output', 'sig_o', 'output_stream_cint16 * restrict', '', '', '', '4*N' }  PortAttrsEnables={'off', 'off', 'off', 'off', 'off', 'off', 'off';'off', 'off', 'off', 'off', 'off', 'off', 'on'}  SampleTime=-1  ClassDeclTypeOptions=C[1 1]@t74@template < unsigned int pattern, unsigned int NSAMP > class polyphase_fir;  ClassDecl=template < unsigned int pattern, unsigned int NSAMP > class polyphase_fir;  ClassTemplateParams={ 'pattern', 'unsigned int', '6'; 'NSAMP', 'unsigned int', '4*N' }  ClassTemplateParamsEnables={'off', 'off', 'on';'off', 'off', 'on'}  ClassCtorDeclTypeOptions=C[1 1]@t69@polyphase_fir(int16 ( & taps0_i ) [ 64 ], int16 ( & taps1_i ) [ 64 ])  ClassCtorDecl=polyphase_fir(int16 ( & taps0_i ) [ 64 ], int16 ( & taps1_i ) [ 64 ])  ClassCtorParams={ 'taps0_i', 'int16 ( &) [ 64 ]', 'tile6_tapsA'; 'taps1_i', 'int16 ( &) [ 64 ]', 'tile6_tapsB' }  KernelHeaderFile=aie/polyphase_fir.h  KernelClassName=polyphase_fir  KernelFunction=run_i  KernelSourceFile=aie/polyphase_fir.cpp  KernelSearchPaths={}  PreProcOptions={}  blockJsonConstraints=[]
      KernelAllAttrs=|
      | s[12;12;9;9;19;14;21;23;21;23;24;21;15;17;12;24;26;26;26;27;28;9;21;23;23;23;24;25;14;19;19;29]@FunctionNameDeclFileNamePortNamesPortTypesPortSerializedTypesPortDirectionsPortWindowSizeEnablesPortWindowMarginEnablesPortBufferSizeEnablesPortBufferMarginEnablesPortSynchronicityEnablesPortSignalSizeEnablesPortBufferSizesPortBufferMarginsFunctionDeclFunctionTemplateSpecKindFunctionTemplateParamNamesFunctionTemplateParamKindsFunctionTemplateParamTypesFunctionTemplateParamValuesFunctionTemplateParamEnablesClassDeclClassTemplateSpecKindClassTemplateParamNamesClassTemplateParamKindsClassTemplateParamTypesClassTemplateParamValuesClassTemplateParamEnablesClassCtorDeclsClassCtorParamNamesClassCtorParamTypesClassCtorParamSerializedTypes[1 1]@C[32 1]@t5@run_it25@../../aie/polyphase_fir.hC[2 1]@t5@sig_it5@sig_oC[2 1]@t30@input_stream_cint16 * restrictt31@output_stream_cint16 * restrictC[2 1]@t37@{Q2{P{Tinput_stream{1{t{Scint16}}}}}}t38@{Q2{P{Toutput_stream{1{t{Scint16}}}}}}C[2 1]@t5@inputt6@outputC[2 1]@l0@l0@C[2 1]@l0@l0@C[2 1]@l0@l0@C[2 1]@l0@l0@C[2 1]@l0@l0@C[2 1]@l0@l1@C[2 1]@nnC[2 1]@nnt158@template < unsigned int pattern, unsigned int NSAMP > 
      | void polyphase_fir::
      | run_i(input_stream_cint16 * restrict sig_i, output_stream_cint16 * restrict sig_o)t4@nonee[0 1]@e[0 1]@e[0 1]@e[0 1]@e[0 1]@t74@template < unsigned int pattern, unsigned int NSAMP > class polyphase_fir;t8@implicitC[2 1]@t7@patternt5@NSAMPC[2 1]@t7@nontypet7@nontypeC[2 1]@t12@unsigned intt12@unsigned intC[2 1]@nnC[2 1]@l1@l1@C[1 1]@t69@polyphase_fir(int16 ( & taps0_i ) [ 64 ], int16 ( & taps1_i ) [ 64 ])C[1 1]@C[2 1]@t7@taps0_it7@taps1_iC[1 1]@C[2 1]@t17@int16 ( &) [ 64 ]t17@int16 ( &) [ 64 ]C[1 1]@C[2 1]@t14@{R{C{Bi16}64}}t14@{R{C{Bi16}64}}
      FunctionDecl=|
      | template < unsigned int pattern, unsigned int NSAMP > 
      | void polyphase_fir::
      | run_i(input_stream_cint16 * restrict sig_i, output_stream_cint16 * restrict sig_o)
  run_i8 : aieBasic/AIE Class Kernel  KernelAllAttrs=|  PortNames={'sig_i'; 'sig_o'}  PortSerializedTypes={'{Q2{P{Tinput_stream{1{t{Scint16}}}}}}'; '{Q2{P{Toutput_stream{1{t{Scint16}}}}}}'}  PortWindowSizes={0.000000000000000000e+00; 0.000000000000000000e+00}  PortWindowMargins={0.000000000000000000e+00; 0.000000000000000000e+00}  PortSynchronicities={'auto', 'auto'}  PortSignalSizes={0.000000000000000000e+00; 2.048000000000000000e+03}  ClassTemplateSpecKind=implicit  ClassTemplateParamNames={'pattern'; 'NSAMP'}  ClassTemplateParamKinds={'nontype'; 'nontype'}  ClassTemplateParamTypes={'unsigned int'; 'unsigned int'}  ClassTemplateParamValues={'7', '2048'}  ClassCtorParamNames={'taps0_i'; 'taps1_i'}  ClassCtorParamSerializedTypes={'{R{C{Bi16}64}}'; '{R{C{Bi16}64}}'}  ClassCtorParamValues={'[-13;54;-178;1985;-20;88;-287;1822;-22;100;-326;1570;-19;93;-307;1256;259;-80;23;-8;569;-166;49;-9;911;-248;74;-14;1256;-307;93;-19;-14;74;-248;911;-9;49;-166;569;-8;23;-80;259;0;2;-4;6;1570;-326;100;-22;1822;-287;88;-20;1985;-178;54;-13;2042;6;-4;2]', '[-6;28;-95;2027;-17;74;-241;1916;-22;97;-314;1706;-21;99;-322;1419;124;-40;12;6;408;-123;36;-8;737;-209;62;-12;1085;-281;85;-17;-17;85;-281;1085;-12;62;-209;737;-8;36;-123;408;6;12;-40;124;1419;-322;99;-21;1706;-314;97;-22;1916;-241;74;-17;2027;-95;28;-6]'}  ClassIndex=1  ClassCtorIndex=1  ClassTabVisible=on  ClassTemplateParamsVisible=on  ClassCtorDeclVisible=on  ClassCtorParamsVisible=on  FunctionTabVisible=on  FunctionDecl=|  PortAttrs={ 'input', 'sig_i', 'input_stream_cint16 * restrict', '', '', '', ''; 'output', 'sig_o', 'output_stream_cint16 * restrict', '', '', '', '4*N' }  PortAttrsEnables={'off', 'off', 'off', 'off', 'off', 'off', 'off';'off', 'off', 'off', 'off', 'off', 'off', 'on'}  SampleTime=-1  ClassDeclTypeOptions=C[1 1]@t74@template < unsigned int pattern, unsigned int NSAMP > class polyphase_fir;  ClassDecl=template < unsigned int pattern, unsigned int NSAMP > class polyphase_fir;  ClassTemplateParams={ 'pattern', 'unsigned int', '7'; 'NSAMP', 'unsigned int', '4*N' }  ClassTemplateParamsEnables={'off', 'off', 'on';'off', 'off', 'on'}  ClassCtorDeclTypeOptions=C[1 1]@t69@polyphase_fir(int16 ( & taps0_i ) [ 64 ], int16 ( & taps1_i ) [ 64 ])  ClassCtorDecl=polyphase_fir(int16 ( & taps0_i ) [ 64 ], int16 ( & taps1_i ) [ 64 ])  ClassCtorParams={ 'taps0_i', 'int16 ( &) [ 64 ]', 'tile7_tapsA'; 'taps1_i', 'int16 ( &) [ 64 ]', 'tile7_tapsB' }  KernelHeaderFile=aie/polyphase_fir.h  KernelClassName=polyphase_fir  KernelFunction=run_i  KernelSourceFile=aie/polyphase_fir.cpp  KernelSearchPaths={}  PreProcOptions={}  blockJsonConstraints=[]
      KernelAllAttrs=|
      | s[12;12;9;9;19;14;21;23;21;23;24;21;15;17;12;24;26;26;26;27;28;9;21;23;23;23;24;25;14;19;19;29]@FunctionNameDeclFileNamePortNamesPortTypesPortSerializedTypesPortDirectionsPortWindowSizeEnablesPortWindowMarginEnablesPortBufferSizeEnablesPortBufferMarginEnablesPortSynchronicityEnablesPortSignalSizeEnablesPortBufferSizesPortBufferMarginsFunctionDeclFunctionTemplateSpecKindFunctionTemplateParamNamesFunctionTemplateParamKindsFunctionTemplateParamTypesFunctionTemplateParamValuesFunctionTemplateParamEnablesClassDeclClassTemplateSpecKindClassTemplateParamNamesClassTemplateParamKindsClassTemplateParamTypesClassTemplateParamValuesClassTemplateParamEnablesClassCtorDeclsClassCtorParamNamesClassCtorParamTypesClassCtorParamSerializedTypes[1 1]@C[32 1]@t5@run_it25@../../aie/polyphase_fir.hC[2 1]@t5@sig_it5@sig_oC[2 1]@t30@input_stream_cint16 * restrictt31@output_stream_cint16 * restrictC[2 1]@t37@{Q2{P{Tinput_stream{1{t{Scint16}}}}}}t38@{Q2{P{Toutput_stream{1{t{Scint16}}}}}}C[2 1]@t5@inputt6@outputC[2 1]@l0@l0@C[2 1]@l0@l0@C[2 1]@l0@l0@C[2 1]@l0@l0@C[2 1]@l0@l0@C[2 1]@l0@l1@C[2 1]@nnC[2 1]@nnt158@template < unsigned int pattern, unsigned int NSAMP > 
      | void polyphase_fir::
      | run_i(input_stream_cint16 * restrict sig_i, output_stream_cint16 * restrict sig_o)t4@nonee[0 1]@e[0 1]@e[0 1]@e[0 1]@e[0 1]@t74@template < unsigned int pattern, unsigned int NSAMP > class polyphase_fir;t8@implicitC[2 1]@t7@patternt5@NSAMPC[2 1]@t7@nontypet7@nontypeC[2 1]@t12@unsigned intt12@unsigned intC[2 1]@nnC[2 1]@l1@l1@C[1 1]@t69@polyphase_fir(int16 ( & taps0_i ) [ 64 ], int16 ( & taps1_i ) [ 64 ])C[1 1]@C[2 1]@t7@taps0_it7@taps1_iC[1 1]@C[2 1]@t17@int16 ( &) [ 64 ]t17@int16 ( &) [ 64 ]C[1 1]@C[2 1]@t14@{R{C{Bi16}64}}t14@{R{C{Bi16}64}}
      FunctionDecl=|
      | template < unsigned int pattern, unsigned int NSAMP > 
      | void polyphase_fir::
      | run_i(input_stream_cint16 * restrict sig_i, output_stream_cint16 * restrict sig_o)
  z0 : Outport
  z1 : Outport  Port=2
  z2 : Outport  Port=3
  z3 : Outport  Port=4
  z4 : Outport  Port=5
  z5 : Outport  Port=6
  z6 : Outport  Port=7
  z7 : Outport  Port=8
  wires:
  run_i6/1 -> z5/1
  run_i1/1 -> z0/1
  x0/1 -> run_i1/1
  run_i4/1 -> z3/1
  run_i2/1 -> z1/1
  x2/1 -> run_i3/1
  x4/1 -> run_i5/1
  x7/1 -> run_i8/1
  run_i8/1 -> z7/1
  x6/1 -> run_i7/1
  run_i3/1 -> z2/1
  x5/1 -> run_i6/1
  x1/1 -> run_i2/1
  x3/1 -> run_i4/1
  run_i5/1 -> z4/1
  run_i7/1 -> z6/1
